simulink model "rti1401_program_nova"  (R2017b)
settings: Solver=ode1  StartTime=0.0  StopTime=Inf  FixedStep=0.001  RelTol=1e-3  EnableMultiTasking=on
PreLoadFcn:
  | dataCar
  | load_vars
  | structAero
  | structEstimPar
  | structSensors
  | structSettings
PostLoadFcn:
  | , if any(exist('dsrtsu_mdlpostloadfcn', 'file') == [2, 3, 6]), try dsrtsu_mdlpostloadfcn('Execute', bdroot); catch fprintf('Error in PostLoadFcn (dsrtsu_mdlpostloadfcn) for model "%s":\n %s\n', bdroot, lasterr); end, end,
InitFcn:
  | dataCar
  | load_vars
  | structAero
  | structEstimPar
  | structSensors
  | structSettings
StartFcn:
  | dataCar
  | load_vars
  | structAero
  | structEstimPar
  | structSensors
  | structSettings
values from neighbouring files (symbols this model uses):
  Throttle_limits = [0.15, 0.90, 0.16, 0.92]    [load_vars.m]
libraries: rtican x44, hdlsllib x32, simulink x8, rti1401lib_II_base x1, fuzblock x1
(part 11 of 11)

== matlab function rti1401_program_nova/Processor/Vehicle Estimated Parameters/Aerodynamic forces ==
  data: aero output Bus: aeroBus =0; v input; car parameter
function aero = aerodynamics(v, car)
aero.FD = 0.5*car.Cd*car.AFront*car.rhoAir*v^2; %drag force, pointing rearward [N]
aero.FL = 0.5*car.Cl*car.AFront*car.rhoAir*v^2; %lift force, pointing upward [N]
aero.lever_FD = [-0.1;0.1]; %distance from the COG to the point of application of the drag [m]
aero.lever_FL = [-0.1;0.1]; %distance from the COG to the point of application of the lift [m]

== matlab function rti1401_program_nova/Processor/Vehicle Estimated Parameters/Efficiency Estimator ==
  data: sensors input; eff output; settings input; car parameter
function eff = Efficiency(sensors,settings,car)
%P_elec * eff = P_mech

persistent effTemp; if isempty(effTemp); effTemp = 0.7; end
persistent errorInt; if isempty(errorInt); errorInt = 0; end

Pmax = car.Pmax - car.PC.safetyMargin; %[W]

P_mech = sum(sensors.torque.*sensors.wheelspeed); %*car.gearRatio
P_elec = sensors.P_elec;
ratio = 0.2;

if settings.effEstimation == 1
    
    if P_elec > 1
        effCalc = P_mech/P_elec;
        effTemp = effTemp*ratio + (1-ratio)*min(max(effCalc,car.PC.minEff),car.PC.maxEff);
        
    elseif P_elec < 1
        effCalc = P_elec/min(P_mech,-1);
        effTemp = effTemp*ratio + (1-ratio)*min(max(effCalc,car.PC.minEff),car.PC.maxEff);
        
        
        %mogelijkheid tot uitbreiding: Pmax variable ifv van batterij voor tijdens
        %indurance
    end
    
end

if settings.effEstimation == 2
    
    if P_elec > Pmax*0.3 && sensors.throttle > 0 % only positive power limit
        
        error = (Pmax - P_elec)/Pmax;
        if error < 0 % P_elec > Pmax
            error = error*2;
        end
        
        errorInt = errorInt + error*car.dt;
        errorInt = max(min(errorInt,0.2),-0.2);
        
        dEff = car.PC.Kp*error + car.PC.Ki*errorInt; %more fitting variable name would be powerReductionFactor as this is not anymore an efficiency as Pelec * eff = Pmech
        %make car.PC.Kp velocity dependend?
        
        effTemp = max(min(effTemp + dEff,car.PC.maxEff),car.PC.minEff);
        
    else
        if P_elec > 5000
            eta = P_mech/P_elec;
            effTemp = effTemp*ratio+(1-ratio)*min(max(eta,car.PC.minEff),car.PC.maxEff);
        elseif P_elec < -5000
            eta = P_elec/min(P_mech,-1);
            effTemp = effTemp*ratio+(1-ratio)*min(max(eta,car.PC.minEff),car.PC.maxEff);
        end
        
    end
    
else
    effTemp = effTemp;
    
end


eff = effTemp;
effnotcontrolled = P_mech/P_elec;

== matlab function rti1401_program_nova/Processor/Vehicle Estimated Parameters/Estim Par ==
  data: v input; estimPar output Bus: estimParBus =0; Fzi input; Fxi input; Fyi input; rref input; mu input; slip input; eff input
function estimPar = fcn(v,Fzi,Fxi,Fyi,rref,mu,slip,eff)

estimPar.v=v;
estimPar.Fzi=Fzi;
estimPar.Fxi=Fxi;
estimPar.Fyi=Fyi;
estimPar.rref=rref;
estimPar.mu=mu;
estimPar.slip=slip;
estimPar.eff=eff;

== matlab function rti1401_program_nova/Processor/Vehicle Estimated Parameters/Fx Estimator  ==
  data: sensors input; Fxi output; v input; car parameter
function Fxi = Fx_Estimator(sensors, v, car)
%OPM: gearratio zit al verwerkt in sensors.torque (= wheelTorque)

persistent wheelspeedPrev; if isempty(wheelspeedPrev); wheelspeedPrev = [0 ;0 ;0 ;0]; end
persistent inertia; if isempty(inertia); inertia = car.tireInertia; end
if isempty(v); v =0;end
wheelspeed = sensors.wheelspeed;
alpha = (wheelspeed - wheelspeedPrev)/car.dt;

%wheelTorque = car.gearRatio*sensors.torque -(car.motor.Inertia*car.gearRatio^2 - car.tireInertia)*alpha;
%to be used if only motor torque is known (real scenario)

%Fxi_est = (wheelTorque - alpha*inertia)/car.tireRadius;
Fxi_est = (sensors.torque - alpha*inertia)/car.tireRadius;
%Fxi_est = (sensors.torque)/car.tireRadius;

Fx_tot = sensors.ax*car.mass + 0.5*car.rhoAir*v^2*car.Cd*car.AFront;
Fxi = Fxi_est;




wheelspeedPrev=wheelspeed;
inertiaOut = inertia;

== matlab function rti1401_program_nova/Processor/Vehicle Estimated Parameters/Fy Estimator  ==
  data: sensors input; Fyi output; Fzi input; Fxi input; car parameter
function Fyi = Fy_Estimator(sensors, Fzi, Fxi, car)

Fyi=[0;0;0;0];
persistent yawRatePrev; if isempty(yawRatePrev); yawRatePrev = sensors.yawRate; end
persistent M_Fx; if isempty(M_Fx); M_Fx = 0; end
persistent M_Fy; if isempty(M_Fy); M_Fy = 0; end
persistent FyRear; if isempty(FyRear); FyRear = 0; end
persistent FzRatioFront; if isempty(FzRatioFront);FzRatioFront = 0; end
persistent FzRatioRear; if isempty(FzRatioRear); FzRatioRear = 0; end
persistent FyFront; if isempty(FyFront); FyFront = 0; end
persistent Fy_FL; if isempty(Fy_FL); Fy_FL = 0; end

scaleFactorFy = 0.7;

yawAcc = (sensors.yawRate - yawRatePrev) * car.fECU;

wheelAngle = (sensors.wheelAngles(1)+sensors.wheelAngles(2))/2;

%Calculate contributions to the moment from lateral forces through the
%total yaw moment and moment of the longitudinal forces.
M_YawTot = car.yawInertia*yawAcc;
M_Fx = (car.tw/2)*cos(wheelAngle)*(Fxi(1)-Fxi(2))...
    +car.lf*sin(wheelAngle)*(Fxi(1)+Fxi(2))...
    +(car.tw/2)*(Fxi(3)-Fxi(4));
M_Fy = M_YawTot - M_Fx;

%Distribution of lateral force on front and rear axle
%NOTE %sin(steerinAngle) deel wordt momenteel verwaarloosd
%     %--> FyFR - FyFL =~ 0
Fy = car.mass*sensors.ay;
FyRear = (cos(wheelAngle)*car.lf*Fy - M_Fy)/...
    (cos(wheelAngle)*car.lf+car.lr);
FyFront = Fy - FyRear;

%Distribution of lateral force on left and right tire by using the normal
%force distribution.

%Use of a scale factor 

FzRatioFront = [Fzi(1); Fzi(2)]./sum(Fzi(1:2));
FzRatioRear = [Fzi(3); Fzi(4)]./sum(Fzi(3:4));



FyFrontDiff = (FzRatioFront(1) - FzRatioFront(2))*scaleFactorFy/2;
Fy_FL = FyFront/2 + FyFrontDiff* FyFront;
Fy_FR = FyFront/2 - FyFrontDiff* FyFront;
FyRearDiff = (FzRatioRear(1) - FzRatioRear(2))*scaleFactorFy/2;
Fy_RL = FyRear/2 + FyRearDiff* FyRear;
Fy_RR = FyRear/2 - FyRearDiff* FyRear;
    
Fyi=[Fy_FL;Fy_FR;Fy_RL;Fy_RR];

yawRatePrev=sensors.yawRate;

== matlab function rti1401_program_nova/Processor/Vehicle Estimated Parameters/Fz Estimator  ==
  data: sensors input; Fzi output; v input; car parameter; aero input
function Fzi = Fz_Estimator(sensors, v,car, aero)
if isempty(v); v =0;end
%Dynamical loads 
%Without taking suspension into account


FFA = car.g*car.mass*car.lr/car.wb - (car.h/car.wb)*(car.mass*sensors.ax) - aero.FD*((car.h+aero.lever_FD(2))/car.wb) - aero.FL*((car.lr-aero.lever_FL(1))/car.wb); %dyn load Front Axle
FRA = car.g*car.mass*car.lf/car.wb + (car.h/car.wb)*(car.mass*sensors.ax) + aero.FD*((car.h+aero.lever_FD(2))/car.wb) - aero.FL*((car.lf+aero.lever_FL(1))/car.wb); %dyn load Rear Axle


FFL = FFA/2 - (car.h/(2*car.tw))*(car.mass*sensors.ay);
FFR = FFA/2 + (car.h/(2*car.tw))*(car.mass*sensors.ay);
FRL = FRA/2 - (car.h/(2*car.tw))*(car.mass*sensors.ay);
FRR = FRA/2 + (car.h/(2*car.tw))*(car.mass*sensors.ay);


Fzi = [FFL;FFR;FRL;FRR];

== matlab function rti1401_program_nova/Processor/Vehicle Estimated Parameters/Mu&Slip Estimator ==
  data: sensors input; mu output; slip output; v input; car parameter
function [mu,slip]= mu_slip(sensors,v,car)

if isempty(v); v =0;end
yawRate = [0;0;sensors.yawRate];
dist = [car.lf   -car.lf   car.lr   -car.lr;
        car.tw/2 -car.tw/2 car.tw/2 -car.tw/2;
        0        0         0        0];
omegaR = sensors.wheelspeed*car.tireRadius;

%Thesis BreyneMeulemans eq 3.20-3.22
v_xcomp = zeros(4,1);
d = sensors.wheelAngles;
for i=1:4
    R = [cos(d(i)) sin(d(i)) 0;
        -sin(d(i)) cos(d(i)) 0;
        0          0         1];
    v_rel = cross(yawRate,dist(:,i));
    v_abs = v_rel + [v;0;0];
    v_ab2 = R*v_abs;
    v_xcomp(i) = v_ab2(1);
end

if sensors.ax > 0
    slip = (omegaR - v_xcomp)./omegaR;
elseif sensors.ax < 0
    slip = (omegaR - v_xcomp)./v_xcomp;
else
    slip = [0;0;0;0];
end

mu = [car.mu;car.mu;car.mu;car.mu];

end

== matlab function rti1401_program_nova/Processor/Vehicle Estimated Parameters/Velocity Estimator/Fuzzy Velocity/FuzzyVelicityGenerator ==
  data: k1 input; vFuzzy output; k2 input; k3 input; k4 input; k5 input; sensors input; settings input; car parameter
function vFuzzy = fuzzyVelocityGenerator(k1,k2,k3,k4,k5,sensors,settings,car)

persistent vFuzzyPrev; if isempty(vFuzzyPrev); vFuzzyPrev = 0; end

beta=0;


vRFL_COG = (sensors.wheelspeed(1)*car.tireRadius...
    + sensors.yawRate*(car.tw/2-car.lf*beta))...
    *cos(sensors.wheelAngles(1)-beta);
vRFR_COG = (sensors.wheelspeed(2)*car.tireRadius...
    - sensors.yawRate*(car.tw/2+car.lf*beta))...
    *cos(sensors.wheelAngles(2)-beta);
vRRL_COG = (sensors.wheelspeed(3)*car.tireRadius...
    + sensors.yawRate*(car.tw/2+car.lr*beta))...
    *cos(beta);
vRRR_COG = (sensors.wheelspeed(4)*car.tireRadius...
    - sensors.yawRate*(car.tw/2-car.lr*beta))...
    *cos(beta);
vR_COG=[vRFL_COG;vRFR_COG;vRRL_COG;vRRR_COG];

vFuzzy = (sum([k1;k2;k3;k4].*vR_COG)+k5*(vFuzzyPrev+car.dt*sensors.ax))...
    /(k1+k2+k3+k4+k5);

vFuzzyPrev = vFuzzy;

== matlab function rti1401_program_nova/Processor/Vehicle Estimated Parameters/Velocity Estimator/Fuzzy Velocity/fuzzyParam ==
  data: sensors input; deltaVFL output; vFuzzyPrev input; deltaVFR output; deltaVRL output; deltaVRR output; maxDeltaV output; car parameter
function [deltaVFL,deltaVFR,deltaVRL,deltaVRR,maxDeltaV]= fuzzyParam(sensors,vFuzzyPrev,car)
beta=0;
vRFL_COG = (sensors.wheelspeed(1)*car.tireRadius...
    + sensors.yawRate*(car.tw/2-car.lf*beta))...
    *cos(sensors.wheelAngles(1)-beta);
vRFR_COG = (sensors.wheelspeed(2)*car.tireRadius...
    - sensors.yawRate*(car.tw/2+car.lf*beta))...
    *cos(sensors.wheelAngles(2)-beta);
vRRL_COG = (sensors.wheelspeed(3)*car.tireRadius...
    + sensors.yawRate*(car.tw/2+car.lr*beta))...
    *cos(beta);
vRRR_COG = (sensors.wheelspeed(4)*car.tireRadius...
    - sensors.yawRate*(car.tw/2-car.lr*beta))...
    *cos(beta);
vR_COG=[vRFL_COG;vRFR_COG;vRRL_COG;vRRR_COG];

deltaVFL = vRFL_COG-vFuzzyPrev;
deltaVFR = vRFR_COG-vFuzzyPrev;
deltaVRL = vRRL_COG-vFuzzyPrev;
deltaVRR = vRRR_COG-vFuzzyPrev;

maxDeltaV = abs(vFuzzyPrev-max(vR_COG))+abs(vFuzzyPrev-min(vR_COG));

== matlab function rti1401_program_nova/Processor/Vehicle Estimated Parameters/Yaw Rate Reference ==
  data: sensors input; rref output; v input; car parameter
function rref = yawRateRef(sensors, v, car)
if isempty(v); v =0;end
%Ackermann
wheelAngle = (sensors.wheelAngles(1)+sensors.wheelAngles(2))/2;
rref = wheelAngle*v/car.wb;

% des_yaw_rate = vx*steering_angle / ...
%     (L_f + L_r + ...
%     m_chassis*vx^2*(L_r*(C_x_alpha_RL+C_x_alpha_RR)-L_f*(C_x_alpha_FL+C_x_alpha_FR))/...
%     ((C_x_alpha_RL+C_x_alpha_RR)*(C_x_alpha_FL+C_x_alpha_FR)*L));

== matlab function rti1401_program_nova/Processor/Sensors ==
  data: ax input; sensors output Bus: sensorBus size=1 =0; ay input; yawRate input; steeringAngle input; steerAngleFL input; steerAngleFR input; throttle input; brake input; wheelspeed_FL input; wheelspeed_FR input; wheelspeed_RL input; wheelspeed_RR input; torqueFL input; torqueFR input; torqueRL input; torqueRR input; P_elec input; car parameter
function sensors = sensors(ax,ay,yawRate,steeringAngle,steerAngleFL,steerAngleFR, throttle,brake,wheelspeed_FL,wheelspeed_FR,wheelspeed_RL,wheelspeed_RR,torqueFL,torqueFR,torqueRL,torqueRR,P_elec,car)

sensors.ax = double(ax);
if ax > 50 || ax < -50
    sensors.ax_error = 1;
else
    sensors.ax_error = 0;
end
sensors.ay = double(ay);
if ay > 50 || ay < -50
    sensors.ay_error = double(1);
else
    sensors.ay_error = double(0);
end

sensors.wheelspeed = double([wheelspeed_FL;wheelspeed_FR;wheelspeed_RL;wheelspeed_RR]);
if wheelspeed_FL > 20000 || wheelspeed_FL < -1000
    sensors.wheelspeed_error = 1;
elseif wheelspeed_FR > 20000 || wheelspeed_FR < -1000
    sensors.wheelspeed_error = 1;
elseif wheelspeed_RL > 20000 || wheelspeed_RL < -1000
    sensors.wheelspeed_error = 1;
elseif wheelspeed_RR > 20000 || wheelspeed_RR < -1000
    sensors.wheelspeed_error = 1;
else
    sensors.wheelspeed_error = 0;
end
sensors.wheelspeed = double(sensors.wheelspeed./60.*2.*pi); %rpm to rad/s

sensors.yawRate = double(yawRate);
if yawRate > 50 || yawRate < -50
    sensors.yawRate_error = 1;
else
    sensors.yawRate_error = double(0);
end

sensors.steerAngle = double(steeringAngle);
if steeringAngle > 300 || steeringAngle < -300
    sensors.steerAngle_error = 1;
else
    sensors.steerAngle_error = double(0);
end

sensors.wheelAngles = double([steerAngleFL;steerAngleFR;0;0]);
if steerAngleFL > 40 || steerAngleFL < -40
    sensors.wheelAngle_error = 1;
elseif steerAngleFR > 40 || steerAngleFR < -40
    sensors.wheelAngle_error = 1;
else
    sensors.wheelAngle_error = 0;
end

sensors.throttle = double(throttle);
if throttle > 100 || throttle < 0
    sensors.throttle_error = double(1);
else
    sensors.throttle_error = 0;
end

sensors.brake = double(brake);
if brake > 100 || brake < 0
    sensors.brake_error = double(1);
else
    sensors.brake_error = 0;
end

sensors.torque = double([torqueFL;torqueFR;torqueRL;torqueRR]);
if torqueFL > 25 || torqueFL < -25
    sensors.torque_error = 1;
elseif torqueFR > 25 || torqueFR < -25
    sensors.torque_error = 1;
elseif torqueRL > 25 || torqueRL < -25
    sensors.torque_error = 1;
elseif torqueRR > 25 || torqueRR < -25
    sensors.torque_error = 1;
else
    sensors.torque_error = 0;
end

sensors.P_elec = double(P_elec);
if P_elec > 160 || P_elec < 0
    sensors.P_elec_error = 1;
else
    sensors.P_elec_error = 0;
end

sensors.errors = [sensors.ax_error;sensors.ay_error;sensors.wheelspeed_error;...
    sensors.yawRate_error;sensors.wheelAngle_error;sensors.throttle_error;...
    sensors.brake_error;sensors.torque_error;sensors.P_elec_error];
sensors.TCRE = [sensors.ax_error;sensors.ay_error;sensors.wheelspeed_error;...
    sensors.throttle_error;sensors.brake_error;sensors.torque_error;...
    sensors.P_elec_error];
    %Traction Control Relevant Errors

AccVector = [sensors.ax;sensors.ay;0]+cross([0;0;sensors.yawRate],...
    [car.distECUx;car.distECUy;car.distECUz])+cross([0;0;sensors.yawRate],...
    cross([0;0;sensors.yawRate],[car.distECUx;car.distECUy;car.distECUz]));
sensors.ax = AccVector(1);
sensors.ay = AccVector(2);
    %Acceleration transformation
    %Thesis BreyneMeulemans eq 3.2

== matlab function rti1401_program_nova/Processor/Ackermann Arno ==
  data: x input; thetaL output; thetaR output
function [thetaL, thetaR]= ackermann(x)
%x is de rack travel in mm
%+ als rack naar rechts beweegt van achter de wagen bekeken
%- als rack naar links beweegt van achter de wagen bekeken

thetaL=-2*(10^-9)*(x^6)+8*(10^-8)*(x^5)+9*(10^-7)*(x^4)+3*(10^-5)*(x^3)-0.0049*(x^2)+1.0437*x+0.0254;
%thetaL is hoeverdraaiing van linker wiel in °
%-hoek is draaien naar links van boven de wagen bekeken
%+hoek is draaien naar rechts van boven de wagen bekeken

thetaR=2*(10^-9)*(x^6)+8*(10^-8)*(x^5)-9*(10^-7)*(x^4)+3*(10^-5)*(x^3)+0.0049*(x^2)+1.0437*x-0.0254;
%thetaR is hoekverdraaiing van rechter wiel in °
%-hoek is draaien naar links van boven de wagen bekeken
%+hoek is draaien naar rechts van boven de wagen bekeken

end
